simulink model "assignment3"  (R2022a)
settings: Solver=FixedStepAuto  StartTime=0.0  StopTime=inf  FixedStep=0.05  RelTol=1e-3
model workspace (MAT data in the model file):
  SL_ROS_VariableLengthArrays_MaxSizes.CommonInfo.ArrayTruncateAction = 'EmitWarning'
  SL_ROS_VariableLengthArrays_MaxSizes.MsgTypeMap = containers.Map
  SL_ROS_VariableLengthArrays_MaxSizes.MsgTypeMap.serialization.keys = {'sensor_msgs/Image'}
  SL_ROS_VariableLengthArrays_MaxSizes.MsgTypeMap.serialization.values{1}(1).PropertyName = 'Data'
  SL_ROS_VariableLengthArrays_MaxSizes.MsgTypeMap.serialization.values{1}(1).DataType = 'uint8'
  SL_ROS_VariableLengthArrays_MaxSizes.MsgTypeMap.serialization.values{1}(1).MaxLength = 921600
  SL_ROS_VariableLengthArrays_MaxSizes.MsgTypeMap.serialization.values{1}(2).PropertyName = 'Encoding'
  SL_ROS_VariableLengthArrays_MaxSizes.MsgTypeMap.serialization.values{1}(2).DataType = 'uint8'
  SL_ROS_VariableLengthArrays_MaxSizes.MsgTypeMap.serialization.values{1}(2).MaxLength = 128
  SL_ROS_VariableLengthArrays_MaxSizes.MsgTypeMap.serialization.uniformity = 0
  SL_ROS_VariableLengthArrays_MaxSizes.MsgTypeMap.serialization.keyType = 'char'
  SL_ROS_VariableLengthArrays_MaxSizes.MsgTypeMap.serialization.valueType = 'any'
values from neighbouring files (symbols this model uses):
  Angular = twist.Angular    [ExampleHelperGazeboSpawnedModel.m]
  Linear = twist.Linear    [ExampleHelperGazeboSpawnedModel.m]
  Point = pose.Position    [ExampleHelperGazeboSpawnedModel.m]
undefined symbols (not defined in the file or in its folder): gray, Rec, SDTV, X, Y
libraries: robotlib x7, visionstatistics x1, visionconversions x1, visiontextngfix x1, simulink x1
settings Model: Creator=raibuntu  LastModifiedBy=isa
settings OptimizationCC: EnhancedBackFolding=on  PassReuseOutputArgsAs=Individual arguments  ZeroExternalMemoryAtStartup=off  ZeroInternalMemoryAtStartup=off  MaxStackSize=64  OptimizeBlockOrder=speed  DifferentSizesBufferReuse=on  OptimizationCustomize=off  EfficientTunableParamExpr=on
settings DebuggingCC: ParameterTunabilityLossMsg=error
settings HardwareCC: ProdBitPerPointer=32  ProdBitPerSizeT=32  ProdBitPerPtrDiffT=32  ProdLargestAtomicFloat=None  ProdIntDivRoundTo=Undefined  ProdEndianess=Unspecified  ProdWordSize=32  ProdHWDeviceType=Generic->Unspecified (assume 32-bit Generic)
settings ModelReferenceCC: EnableRefExpFcnMdlSchedulingChecks=off
settings SFSimCC: MATLABDynamicMemAlloc=off
settings RTWCC: SystemTargetFile=ert.tlc  HardwareBoard=Robot Operating System (ROS)  TLCOptions="-aInlineSetEventsForThisBaseRateFcn=TLC_FALSE -aSuppressMultiTaskScheduler=TLC_FALSE  -aRateBasedStepFcn=0"  TemplateMakefile=ert_default_tmf  Toolchain=Catkin  TargetLang=C++
settings CodeAppCC: ForceParamTrailComments=on  IgnoreCustomStorageClasses=off  OperatorAnnotations=on  SimulinkDataObjDesc=on  SFDataObjDesc=on  InsertBlockDesc=on

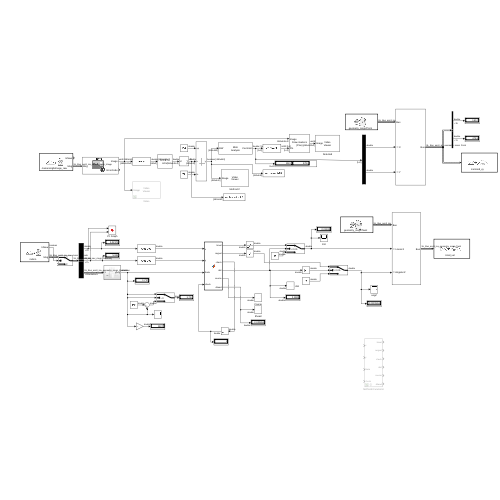
[thumbnail: Simulink's stored preview of the top-level diagram]
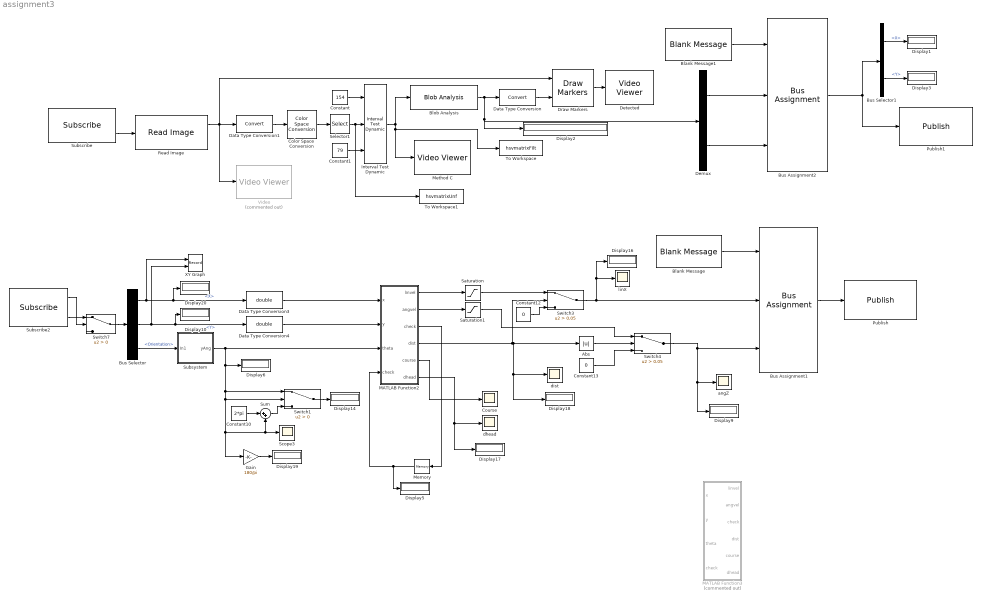
== system assignment3 ==
  Abs : Abs  SaturateOnIntegerOverflow=off
  Blank Message : robotlib/Blank Message  messageClass=Message  entityType=geometry_msgs/Twist  messageType=geometry_msgs/Twist  SampleTime=inf  legacyBusStruct=off
  Blank Message1 : robotlib/Blank Message  messageClass=Message  entityType=geometry_msgs/Point  messageType=geometry_msgs/Point  SampleTime=inf  legacyBusStruct=off
  Blob Analysis : visionstatistics/Blob Analysis  Tag=vipblks_row_conv  area=off  centroid=on  bBox=off  majorAxis=off  minorAxis=off  angle=off  eccentricity=off  equivDiameterSq=off  extent=off  perimeter=off  outDT=double  conn=8  isLabel=off  maxBlobs=1  warnIfNumBlobsExceeded=on  isCount=off  useMinArea=off  minArea=0  useMaxArea=off  maxArea=intmax('uint32')  excludeBorderBlob=off  isOutVarDim=off  isFill=on  fillValues=-1  roundingMode=Floor  overflowMode=off  prodOutputMode=Binary point scaling  prodOutputWordLength=32  prodOutputFracLength=16  accumMode=Binary point scaling  accumWordLength=32  accumFracLength=0  outputMode=Binary point scaling  outputWordLength=32  outputFracLength=16  firstCoeffMode=Binary point scaling  firstCoeffWordLength=16  firstCoeffFracLength=14  secondCoeffMode=Binary point scaling  secondCoeffWordLength=32  secondCoeffFracLength=16
  Bus Assignment1 : BusAssignment  AssignedSignals=Linear.X,Angular.Z
  Bus Assignment2 : BusAssignment  AssignedSignals=X,Y
  Bus Selector : BusSelector  OutputSignals=Pose.Pose.Position.X,Pose.Pose.Position.Y,Pose.Pose.Orientation
  Bus Selector1 : BusSelector  OutputSignals=X,Y
  Color Space Conversion : visionconversions/Color Space  Conversion  conversion=Obsolete  conversionActive=R'G'B' to HSV  wp_str=D65  rec=Rec. 601 (SDTV)  sys=1125/60/2:1  imagePorts=One multidimensional signal
  Constant : Constant  Value=154
  Constant1 : Constant  Value=79
  Constant10 : Constant  Value=2*pi
  Constant12 : Constant  Value=0
  Constant13 : Constant  Value=0
  Course : Scope
  Data Type Conversion : DataTypeConversion  SaturateOnIntegerOverflow=off  RndMeth=Floor
  Data Type Conversion1 : DataTypeConversion  SaturateOnIntegerOverflow=off  RndMeth=Floor
  Data Type Conversion3 : DataTypeConversion  OutDataTypeStr=double  SaturateOnIntegerOverflow=off  RndMeth=Floor
  Data Type Conversion4 : DataTypeConversion  OutDataTypeStr=double  SaturateOnIntegerOverflow=off  RndMeth=Floor
  Demux : Demux  Outputs=2
  Detected : VideoViewer  colormapValue=gray(256)  FigPos=[73 706 956 540]
  Display{1..3,5..6,9..10,14,16..20} (13 alike) : Display
  Draw Markers : visiontextngfix/Draw Markers  shape=Plus  size=30  fill=off  fillClrSource=Specify via dialog  display=User-specified value  intensity=200  color=[255 0 0]  opacity=0.6  viewport=Entire image  antialiasing=off  inType=Obsolete  imagePorts=One multidimensional signal  roundingMode=Floor  overflowMode=off  memoryMode=Specify word length  memoryWordLength=16  memoryFracLength=15  prodOutputMode=Binary point scaling  prodOutputWordLength=32  prodOutputFracLength=14
      settings: SourceProductBaseCode=VP
  Gain : Gain  Gain=180/pi
  Interval Test Dynamic : simulink/Logic and Bit Operations/Interval Test Dynamic  IntervalClosedRight=on  IntervalClosedLeft=on  OutDataTypeStr=boolean
      settings: SourceProductBaseCode=SL
  MATLAB Function2 : MATLAB Function  TreatAsAtomicUnit=on
  MATLAB Function3 : Subsystem  Commented=on
      mask help: Simulink:masks:GenSFuncDesc_MD
      mask Help: eval('feval(''rtwprivate'',''rtwhelpview'',''rtw_sfcn_block'')');
  Memory : Memory
  Method C : VideoViewer  colormapValue=gray(256)  FigPos=[73 715 956 563]
  Publish : robotlib/Publish  topicSource=Select from ROS network  topic=/cmd_vel  messageType=geometry_msgs/Twist  legacyBusStruct=off  messageQueueLength=1
  Publish1 : robotlib/Publish  topicSource=Specify your own  topic=/centroid_xy  messageType=geometry_msgs/Point  legacyBusStruct=off  messageQueueLength=1
  Read Image : robotlib/Read Image  MaximumImageSize=[480, 640]  ImageEncoding=rgb8  ShowAlphaOutput=off  ShowErrorCodeOutput=on  VariableSizeOutputs=off
      settings: SourceProductBaseCode=RR
  Saturation : Saturate  UpperLimit=0.2  LowerLimit=-0.2
  Saturation1 : Saturate  UpperLimit=0.4  LowerLimit=-0.4
  Scope3 : Scope
  Selector1 : Selector  NumberOfDimensions=3  InputPortWidth=3  IndexOptions=Index vector (dialog),Index vector (dialog),Index vector (dialog)  Indices=[1:480],[1:640],[3]  OutputSizes=1,1,1
  Subscribe : robotlib/Subscribe  topicSource=Select from ROS network  topic=/camera/rgb/image_raw  messageType=sensor_msgs/Image  SampleTime=-1  legacyBusStruct=off  messageQueueLength=1
  Subscribe2 : robotlib/Subscribe  topicSource=Specify your own  topic=/odom  messageType=nav_msgs/Odometry  SampleTime=-1  legacyBusStruct=off  messageQueueLength=1
  Subsystem : Subsystem
  Sum : Sum  Inputs=|++
  Switch1 : Switch  Criteria=u2 > Threshold  SaturateOnIntegerOverflow=off  InputSameDT=off
  Switch3 : Switch  Criteria=u2 > Threshold  Threshold=0.05  SaturateOnIntegerOverflow=off  InputSameDT=off
  Switch4 : Switch  Criteria=u2 > Threshold  Threshold=0.05  SaturateOnIntegerOverflow=off  InputSameDT=off
  Switch7 : Switch  Criteria=u2 > Threshold  SaturateOnIntegerOverflow=off  InputSameDT=off
  To Workspace : ToWorkspace  VariableName=hsvmatrixFilt  SampleTime=-1
  To Workspace1 : ToWorkspace  VariableName=hsvmatrixUnf  SampleTime=-1
  Video : VideoViewer  Commented=on  colormapValue=gray(256)  FigPos=[78 939 1838 794]
  XY Graph : Record  FileSettingsInternal="{\"entries\":[{\"content\":{\"excelSettings\":{\"content\":{},\"type\":\"Streamout.ExcelSettings\"}},\"type\":\"Streamout.FileSettingStorage\",\"uuid\":\"f44344bb-7819-46ac-a6d0-15586ce5522e\"}],\"packageUris\":[\"http://schema.mathworks.com/mf0/streamout_blocks/R2020a\"],\"version\":\"1.0\"}"  Layout=[1 1]  SignalsInternal="{\"entries\":[{\"content\":{\"signals\":[{\"content\":{\"blockPath\":[\"ass3_isa/XY Graph\"],\"channel\":[],\"dimensions\":[1],\"domain\":\"ass3_isa/XY Graph\",\"lineColor\":\"#edb120\",\"plots\":[],\"port\":1,\"sid\":[\"\"],\"signalID\":20,\"signalName\":\"<X>\"},\"type\":\"RecordBlkView.Signal\",\"uuid\":\"8ec07af6-3c9d-4e8e-8eb6-888bf07ceb31\"},{\"content\":{\"blockPath\":[\"ass3_isa/XY Graph\"],\"channel\":[],\"dimensions\":[1],\"domain\":\"ass3_isa/XY Graph\",\"lineColor\":\"#7e2f8e\",\"plots\":[],\"port\":2,\"sid\":[\"\"],\"signalID\":24,\"signalName\":\"<Y>\"},\"type\":\"RecordBlkView.Signal\",\"uuid\":\"ef94b46a-f6db-4cef-baab-ffb952dc2111\"}]},\"type\":\"RecordBlkView.InputSignals\",\"uuid\":\"994f90ca-2721-4957-ade0-ebeca750b3c4\"}],\"packageUris\":[\"http://schema.mathworks.com/mf0/streamout_blocks/R2020a\"],\"version\":\"1.0\"}"  VisualizationBindings="{\"xyplotplugin\":{\"info\":[{\"series\":[],\"subplotID\":1}]}}"  CompatibilityTag=XY  st=-1
  angZ : Scope
  dhead : Scope
  dist : Scope
  linX : Scope
  wires:
  Draw Markers/1 -> Detected/1
  Data Type Conversion/1 -> Draw Markers/2
  Color Space Conversion/1 -> Selector1/1
  Data Type Conversion1/1 -> Color Space Conversion/1
  Subscribe/2 -> Read Image/1
  Constant/1 -> Interval Test Dynamic/1
  Constant1/1 -> Interval Test Dynamic/3
  Interval Test Dynamic/1 -> Blob Analysis/1, To Workspace/1, Method C/1
  Blob Analysis/1 -> Demux/1, Display2/1, Data Type Conversion/1
  Subscribe2/1 -> Switch7/2
  Blank Message/1 -> Bus Assignment1/1
  Data Type Conversion4/1 -> MATLAB Function2/2(y)
  MATLAB Function2/4(dist) -> Abs/1, Display18/1, dist/1, Switch3/2
  Switch7/1 -> Bus Selector/1
  Abs/1 -> Switch4/2
  MATLAB Function2/5(course) -> Course/1
  Switch1/1 -> Display14/1
  Bus Assignment1/1 -> Publish/1
  Sum/1 -> Switch1/3
  Saturation/1 -> Switch3/1
  Saturation1/1 -> Switch4/1
  Constant10/1 -> Sum/1
  MATLAB Function2/1(linvel) -> Saturation/1
  Gain/1 -> Display19/1
  Switch3/1 -> Display16/1, linX/1, Bus Assignment1/2
  Switch4/1 -> Display9/1, angZ/1, Bus Assignment1/3
  Subscribe2/2 -> Switch7/1
  MATLAB Function2/6(dhead) -> dhead/1, Display17/1
  Constant13/1 -> Switch4/3
  MATLAB Function2/2(angvel) -> Saturation1/1
  Data Type Conversion3/1 -> MATLAB Function2/1(x)
  Constant12/1 -> Switch3/3
  Subsystem/1(yAng) -> MATLAB Function2/3(theta), Display6/1, Switch1/1, Scope3/1, Sum/2, Gain/1, Switch1/2
  Bus Selector/3 -> Subsystem/1(In1)  "<Orientation>"
  Bus Selector/2 -> Data Type Conversion4/1, Display10/1, XY Graph/2  "<Y>"
  Bus Selector/1 -> Data Type Conversion3/1, Display20/1, XY Graph/1  "<X>"
  MATLAB Function2/3(check) -> Memory/1
  Memory/1 -> MATLAB Function2/4("check "), Display5/1
  Read Image/1 -> Data Type Conversion1/1, Draw Markers/1, Video/1
  Selector1/1 -> To Workspace1/1, Interval Test Dynamic/2
  Blank Message1/1 -> Bus Assignment2/1
  Demux/2 -> Bus Assignment2/3
  Demux/1 -> Bus Assignment2/2
  Bus Assignment2/1 -> Publish1/1, Bus Selector1/1
  Bus Selector1/1 -> Display1/1  "<X>"
  Bus Selector1/2 -> Display3/1  "<Y>"

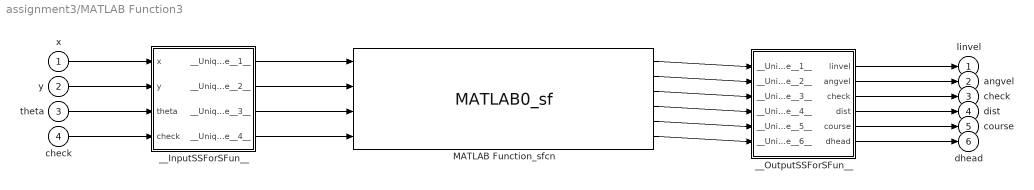
== system assignment3/MATLAB Function3 ==
  x : Inport
  y : Inport  Port=2
  theta : Inport  Port=3
  "check " : Inport  Port=4
  MATLAB Function_sfcn : S-Function  FunctionName=MATLAB0_sf  SFunctionModules=""  SFunctionDeploymentMode=off  EnableBusSupport=off  mask{rtw_sf_name=MATLAB0_sf, showVar=off}
      mask prompts: rtw_sf_name "Simulink:masks:GenSFuncName_MP"; showVar "Simulink:masks:GenSFuncShowModuleList_MP"
      mask help: Simulink:masks:GenSFuncDesc_MD
      mask init:
      | displist = '';
      | if ~strcmp(get_param(gcb, 'FunctionName'), rtw_sf_name);
      |   set_param(gcb, 'FunctionName', rtw_sf_name);
      | end
      | % Check if we are generating code
      | rtw_mode = false;
      | if strcmpi(get_param(bdroot(gcb),'SimulationStatus'),'Initializing')
      | 	rtw_mode = strcmpi(get_param(bdroot(gcb),'BuildingRTWCode'),'on') && ...
      | 		~strcmpi(get_param(bdroot(gcb),'TargetStyle'),'SimulationTarget');
      | end
      | if showVar || rtw_mode
      | 	if exist('rtwsfunc') == 2 | exist('rtwsfunc') == 6
      | 		tmplist = rtwsfunc(rtw_sf_name,gcb);
      | 		tmplist = DAStudio.message('Simulink:masks:GenSFuncListOfModules_IC', tmplist);
      | 	elseif showVar
      | 		tmplist1 = DAStudio.message('Simulink:masks:GenSFuncListOfModules_IC', '');
      |         tmplist2 = DAStudio.message('Simulink:masks:GenSFuncNotLicensed_IC');
      |         tmplist = [tmplist1 tmplist2];
      |  	end
      | end
      | if showVar
      |   displist = tmplist;
      | end
      settings: CopyFcn=|
      | if ~strcmp(get_param(gcb,'Linkstatus'),'none') && ...
      | ~strcmp(get_param(gcb,'Linkstatus'),'implicit')
      |   set_param(gcb,'LinkStatus','none');
      | end
      mask Help: eval('feval(''rtwprivate'',''rtwhelpview'',''rtw_sfcn_block'')');
      mask Display:
      | port_label('input',1,'x');
      | port_label('input',2,'y');
      | port_label('input',3,'theta');
      | port_label('input',4,'check ');
      | port_label('output',1,'linvel');
      | port_label('output',2,'angvel');
      | port_label('output',3,'check');
      | port_label('output',4,'dist');
      | port_label('output',5,'course');
      | port_label('output',6,'dhead');
  __InputSSForSFun__ : Subsystem
  __OutputSSForSFun__ : Subsystem
  linvel : Outport
  angvel : Outport  Port=2
  check : Outport  Port=3
  dist : Outport  Port=4
  course : Outport  Port=5
  dhead : Outport  Port=6
  wires:
  __OutputSSForSFun__/6(dhead) -> dhead/1
  __OutputSSForSFun__/5(course) -> course/1
  __OutputSSForSFun__/4(dist) -> dist/1
  __OutputSSForSFun__/3(check) -> check/1
  __OutputSSForSFun__/2(angvel) -> angvel/1
  __OutputSSForSFun__/1(linvel) -> linvel/1
  MATLAB Function_sfcn/6 -> __OutputSSForSFun__/6(__UniqueInportName__6__)
  MATLAB Function_sfcn/5 -> __OutputSSForSFun__/5(__UniqueInportName__5__)
  MATLAB Function_sfcn/4 -> __OutputSSForSFun__/4(__UniqueInportName__4__)
  MATLAB Function_sfcn/3 -> __OutputSSForSFun__/3(__UniqueInportName__3__)
  MATLAB Function_sfcn/2 -> __OutputSSForSFun__/2(__UniqueInportName__2__)
  MATLAB Function_sfcn/1 -> __OutputSSForSFun__/1(__UniqueInportName__1__)
  __InputSSForSFun__/4(__UniqueOutportName__4__) -> MATLAB Function_sfcn/4
  __InputSSForSFun__/3(__UniqueOutportName__3__) -> MATLAB Function_sfcn/3
  __InputSSForSFun__/2(__UniqueOutportName__2__) -> MATLAB Function_sfcn/2
  __InputSSForSFun__/1(__UniqueOutportName__1__) -> MATLAB Function_sfcn/1
  "check "/1 -> __InputSSForSFun__/4("check ")
  theta/1 -> __InputSSForSFun__/3(theta)
  y/1 -> __InputSSForSFun__/2(y)
  x/1 -> __InputSSForSFun__/1(x)

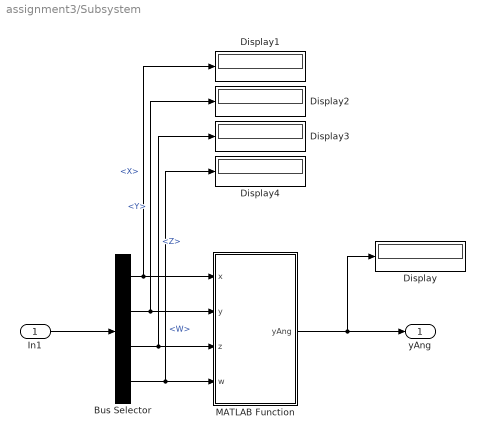
== system assignment3/Subsystem ==
  In1 : Inport
  Bus Selector : BusSelector  OutputSignals=X,Y,Z,W
  Display{,1..4} (5 alike) : Display
  MATLAB Function : MATLAB Function  TreatAsAtomicUnit=on
  yAng : Outport
  wires:
  In1/1 -> Bus Selector/1
  MATLAB Function/1(yAng) -> Display/1, yAng/1
  Bus Selector/2 -> Display2/1, MATLAB Function/2(y)  "<Y>"
  Bus Selector/1 -> MATLAB Function/1(x), Display1/1  "<X>"
  Bus Selector/3 -> Display3/1, MATLAB Function/3(z)  "<Z>"
  Bus Selector/4 -> Display4/1, MATLAB Function/4(w)  "<W>"

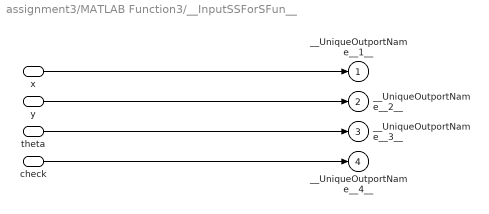
== system assignment3/MATLAB Function3/__InputSSForSFun__ ==
  x : Inport
  y : Inport  Port=2
  theta : Inport  Port=3
  "check " : Inport  Port=4
  __UniqueOutportName__1__ : Outport
  __UniqueOutportName__2__ : Outport  Port=2
  __UniqueOutportName__3__ : Outport  Port=3
  __UniqueOutportName__4__ : Outport  Port=4
  wires:
  "check "/1 -> __UniqueOutportName__4__/1
  theta/1 -> __UniqueOutportName__3__/1
  y/1 -> __UniqueOutportName__2__/1
  x/1 -> __UniqueOutportName__1__/1

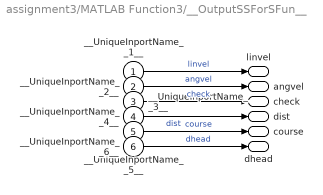
== system assignment3/MATLAB Function3/__OutputSSForSFun__ ==
  __UniqueInportName__1__ : Inport
  __UniqueInportName__2__ : Inport  Port=2
  __UniqueInportName__3__ : Inport  Port=3
  __UniqueInportName__4__ : Inport  Port=4
  __UniqueInportName__5__ : Inport  Port=5
  __UniqueInportName__6__ : Inport  Port=6
  linvel : Outport
  angvel : Outport  Port=2
  check : Outport  Port=3
  dist : Outport  Port=4
  course : Outport  Port=5
  dhead : Outport  Port=6
  wires:
  __UniqueInportName__6__/1 -> dhead/1  "dhead"
  __UniqueInportName__5__/1 -> course/1  "course"
  __UniqueInportName__4__/1 -> dist/1  "dist"
  __UniqueInportName__3__/1 -> check/1  "check"
  __UniqueInportName__2__/1 -> angvel/1  "angvel"
  __UniqueInportName__1__/1 -> linvel/1  "linvel"

== matlab function assignment3/MATLAB Function2 ==
  data: x input; linvel output; y input; theta input; angvel output; check output; dist output; course output; dhead output; check input
function [linvel,angvel,check,dist,course,dhead] = fcn(x,y,theta,check)
wpx     = 0; 
wpy     = 6;
ang     = pi/2;
dist    = sqrt((x - wpx)^2 + (y - wpy)^2);
course  = atan2(wpy - y,wpx - x);
kpv     = 0.2;
kpw     = 0.2;

    if check == 0 
        dhead  = ang - theta;
        if dhead <= 0.03
            check = 1;
            linvel = 0;
            angvel = 0;
        else 
            linvel = 0;
            angvel = kpw*dhead;
            check = 0;
        end
    else
        dhead0 = course - theta;
        if dhead0 < -pi
            dhead = dhead0 + 2*pi;
        elseif dhead0 > pi
            dhead = dhead0 - 2*pi;
        else
            dhead = dhead0;
        end
        linvel  = kpv*dist;
        angvel  = kpw*dhead;
        check   = 1;
    end

end

== matlab function assignment3/Subsystem/MATLAB Function ==
  data: x input; yAng output; y input; z input; w input
function yAng = conversAngle(x,y,z,w)
eulAngle = quat2eul([w,x,y,z]);
yAng = eulAngle(1);
check = isnan(yAng);
if check == 1
    yAng = 0;
end
end
